simulink model "cable_test"  (R2020a)
settings: Solver=VariableStepAuto  StartTime=0.0  StopTime=inf  RelTol=1e-3
libraries: simulink x1, SG_library x1
settings Model: Creator=padlewsk  LastModifiedBy=padlewsk

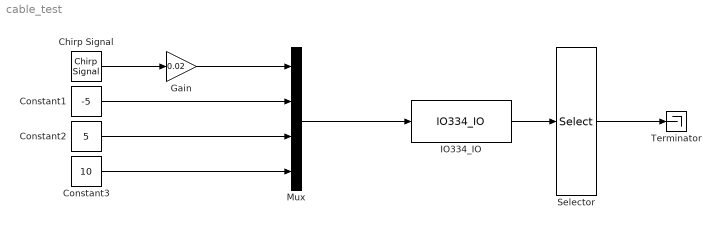
== system cable_test ==
  Chirp Signal : simulink/Sources/Chirp Signal  f1=150  T=20  f2=1500
  Constant1 : Constant  Value=-5
  Constant2 : Constant  Value=5
  Constant3 : Constant  Value=10  SampleTime=-1
  Gain : Gain  Gain=0.02
  IO334_IO : SG_library/Built elements/IO334_IO  ts=20e-6  OutputRange=Auto (same as ADC)
      settings: SourceProductName=Custom Speedgoat implementations
  Mux : Mux
  Selector : Selector  InputPortWidth=16  IndexOptions=Index vector (dialog)  Indices=[5:8]  OutputSizes=1
  Terminator : Terminator
  wires:
  Mux/1 -> IO334_IO/1
  IO334_IO/1 -> Selector/1
  Chirp Signal/1 -> Gain/1
  Constant1/1 -> Mux/2
  Constant2/1 -> Mux/3
  Constant3/1 -> Mux/4
  Gain/1 -> Mux/1
  Selector/1 -> Terminator/1
